simulink library "setTargetPathLoc_ul"  (R2020a)
settings: Solver=VariableStepAuto  StartTime=0.0  StopTime=10.0  RelTol=1e-3
libraries: calcNormalizedPathCoord_ul x1
settings Model: Creator=Ayaz  LastModifiedBy=Ayaz

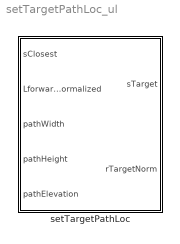
== system setTargetPathLoc_ul ==
  setTargetPathLoc : Subsystem

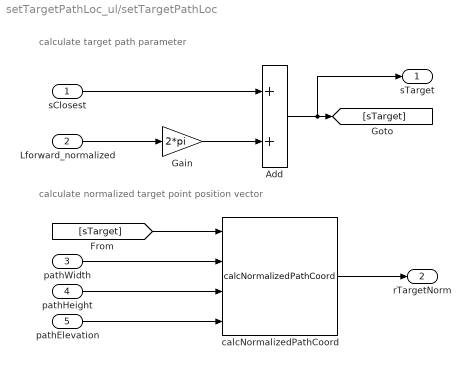
== system setTargetPathLoc_ul/setTargetPathLoc ==
  note: calculate normalized target point position vector
  note: calculate target path parameter
  sClosest : Inport
  Lforward_normalized : Inport  Port=2
  pathWidth : Inport  Port=3
  pathHeight : Inport  Port=4
  pathElevation : Inport  Port=5
  Add : Sum
  Gain : Gain  Gain=2*pi
  calcNormalizedPathCoord : calcNormalizedPathCoord_ul/calcNormalizedPathCoord  SystemSampleTime=-1  Latency=0  AutoFrameSizeCalculation=off
  sTarget : Outport
  rTargetNorm : Outport  Port=2
  wires:
  Lforward_normalized/1 -> Gain/1
  sClosest/1 -> Add/1
  Gain/1 -> Add/2
  Add/1 -> sTarget/1, [sTarget]
  [sTarget] -> calcNormalizedPathCoord/1
  pathElevation/1 -> calcNormalizedPathCoord/4
  pathWidth/1 -> calcNormalizedPathCoord/2
  pathHeight/1 -> calcNormalizedPathCoord/3
  calcNormalizedPathCoord/1 -> rTargetNorm/1
